simulink model "DCMotor2"  (R2023b)
settings: Solver=VariableStepAuto  StartTime=0.0  StopTime=5  RelTol=1e-3
values from neighbouring files (symbols this model uses):
  b = 0.2    [closed_step.m]    (also in low_pass.m; open_step.m)
  J = 0.1    [closed_step.m]    (also in low_pass.m; open_step.m)
  K = 0.02    [closed_step.m]    (also in low_pass.m; open_step.m)
  L = 0.4    [closed_step.m]    (also in low_pass.m; open_step.m)
  R = 2    [closed_step.m]    (also in low_pass.m; open_step.m)
libraries: simulink x1
settings Model: Creator=user  LastModifiedBy=user

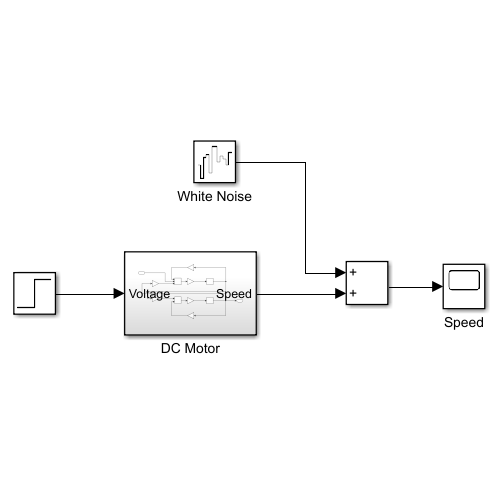
[thumbnail: Simulink's stored preview of the top-level diagram]
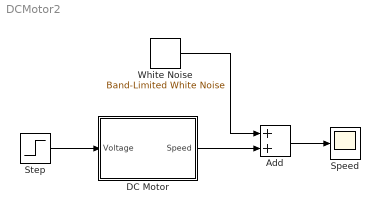
== system DCMotor2 ==
  Add : Sum
  DC Motor : Subsystem
  Speed : Scope
  Step : Step  Time=0  SampleTime=0
  White Noise : simulink/Sources/Band-Limited White Noise  Cov=[0.0000001]  Ts=0.001  seed=1
  wires:
  Step/1 -> DC Motor/1(Voltage)
  DC Motor/1(Speed) -> Add/2
  White Noise/1 -> Add/1
  Add/1 -> Speed/1

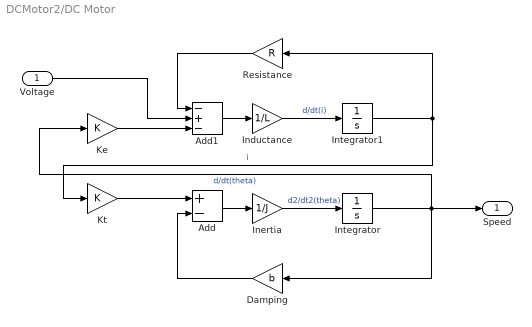
== system DCMotor2/DC Motor ==
  Voltage : Inport
  Add : Sum  Inputs=+-
  Add1 : Sum  Inputs=-+-
  Damping : Gain  Gain=b
  Inductance : Gain  Gain=1/L
  Inertia : Gain  Gain=1/J
  Integrator : Integrator
  Integrator1 : Integrator
  Ke : Gain  Gain=K
  Kt : Gain  Gain=K
  Resistance : Gain  Gain=R
  Speed : Outport
  wires:
  Integrator/1 -> Speed/1, Ke/1, Damping/1  "d/dt(theta)"
  Ke/1 -> Add1/3
  Add1/1 -> Inductance/1
  Resistance/1 -> Add1/1
  Voltage/1 -> Add1/2
  Inductance/1 -> Integrator1/1  "d/dt(i)"
  Integrator1/1 -> Resistance/1, Kt/1  "i"
  Add/1 -> Inertia/1
  Kt/1 -> Add/1
  Inertia/1 -> Integrator/1  "d2/dt2(theta)"
  Damping/1 -> Add/2
